simulink model "spec_Ventilation"  (R2016b)
settings: Solver=VariableStepDiscrete  StartTime=0  StopTime=100  MaxStep=1  RelTol=1e-3  EnableMultiTasking=on
libraries: carnot x6, simulink x1
settings Model: Creator=drhf  LastModifiedBy=drhf
settings DataIOCC: SaveFormat=Array  SignalLoggingSaveFormat=ModelDataLogs
settings OptimizationCC: ExpressionDepthLimit=2147483647  LifeSpan=inf
settings DebuggingCC: UnderspecifiedInitializationDetection=Classic  MergeDetectMultiDrivingBlocksExec=none  SolverPrmCheckMsg=warning  FcnCallInpInsideContextMsg=warning  StateNameClashWarn=warning  SFUnexpectedBacktrackingDiag=warning  SFNoUnconditionalDefaultTransitionDiag=warning  SFExecutionAtInitializationDiag=none
settings HardwareCC: ProdBitPerPointer=32  ProdBitPerSizeT=32  ProdBitPerPtrDiffT=32  ProdLargestAtomicFloat=None  ProdIntDivRoundTo=Undefined  ProdEndianess=Unspecified  ProdWordSize=32  ProdHWDeviceType=32-bit Generic
settings ModelReferenceCC: PropagateSignalLabelsOutOfModel=off
settings GRTTargetCC: TargetLangStandard=C89/C90 (ANSI)  GeneratePreprocessorConditionals=Disable all  CombineOutputUpdateFcns=off  GRTInterface=on
settings ConfigComp: CovMetricSettings=dw  CovHtmlReporting=on  CovSaveCumulativeToWorkspaceVar=on  CovSaveSingleToWorkspaceVar=on  CovExternalEMLEnable=off

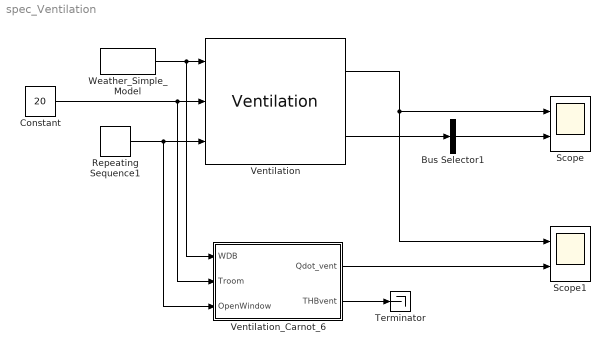
== system spec_Ventilation ==
  Bus Selector1 : BusSelector  OutputSignals=MassFlow  OutputAsBus=on
  Constant : Constant  Value=20
  Repeating Sequence1 : simulink/Sources/Repeating Sequence  rep_seq_t=[0 20 30 60 70 100]  rep_seq_y="[0  0  1   1   0   0]"
  Scope : Scope  NumInputPorts=2
  Scope1 : Scope  NumInputPorts=2
  Terminator : Terminator
  Ventilation : carnot/Source/Ventilation/Ventilation  Ahabit=50  Hroom=2  vent=0.5  rec=0.5  ppmCO2=400  ppmVOC=0  alpha=10  H=1  W=1  Nwin=1
  Ventilation_Carnot_6 : Subsystem  mask(Ventilation with Heat Recovery and Window){Ahabit=50, Hroom=2, vent=0.5, rec=0.5, ppmCO2=400, ppmVOC=0, alpha=10, H=1.2, W=1, Nwin=4}
      mask prompts: Ahabit "A: heated surface of the house in m²"; Hroom "H: height of room in m"; vent "Air exchange rate (volume of house per hour) in 1/h"; rec "Heat recovery of ventilation in 0..1"; ppmCO2 "Concentration of CO2 in ppm"; ppmVOC "Concentration of VOC in ppm"; alpha "maximal opening angle (°)"; H "height of window (m)"; W "width of window (m)"; Nwin "Number of windows"
      mask help:
      | Model of a mechanical ventilation system with heat recovery and a ventilation with windows.
      | The model is suitable for the simple building model (/Load/Houses/House_simpe).
      mask init:
      | rec = max(0, min(1, rec));
      mask Help: web(fullfile(path_carnot('help'),'Ventilation.html'),'-helpbrowser')
      mask TypeOptions Ahabit: Ahabit/Value
      mask TypeOptions Hroom: Hroom/Gain
      mask TypeOptions vent: air_flow_rate/Gain | air_flow_rate1/Gain
      mask TypeOptions rec: heatRecovery/Value
      mask TypeOptions ppmCO2: ppmCO2/Value
      mask TypeOptions ppmVOC: ppmVOC/Value
      mask TypeOptions alpha: Window_Ventilation/alpha
      mask TypeOptions H: Window_Ventilation/H
      mask TypeOptions W: Window_Ventilation/W
      mask TypeOptions Nwin: Window_Ventilation/Nwin
      mask Display:
      | plot(0,-0.2,1.2,1.2,[0.2 0.35], [0.8 0.7])
      | plot([0.35 0.65], [0.7 0.7])
      | plot([0.65 0.8], [0.7 0.8])
      | plot([0.65 0.8], [0.76 0.8])
      | plot([0.7 0.8], [0.65 0.8])
      | 
      | plot([0.2 0.35], [0.2 0.3])
      | plot([0.35 0.65], [0.3 0.3])
      | plot([0.65 0.8], [0.3 0.2])
      | plot([0.2 0.25], [0.2 0.32])
      | plot([0.2 0.35], [0.2 0.23])
      | 
      | plot ([0.45 0.45], [0 1])
      | plot ([0.55 0.55], [0 1])
      | 
      | plot ([0.45 0.55], [0.2 0.2])
      | plot ([0.45 0.55], [0.8 0.8])
      | 
      | plot ([0.45 0.55], [0 0.2])
      | plot ([0.45 0.55], [0.8 1])
  Weather_Simple_Model : carnot/Weather/Weather_Simple_Model  lat=60  Ibn=900  Idg=100  tamb=0  deltaTsky=-6  rh=50  precip="10e-3/24/3600           % 10 mm in 24 h"  cloud=0.125  p=1013e2  vw=1  wdir=270
  wires:
  Ventilation/1 -> Scope1/1, Scope/1
  Constant/1 -> Ventilation_Carnot_6/2(Troom), Ventilation/2
  Repeating Sequence1/1 -> Ventilation_Carnot_6/3(OpenWindow), Ventilation/3
  Ventilation/2 -> Bus Selector1/1
  Weather_Simple_Model/1 -> Ventilation_Carnot_6/1(WDB), Ventilation/1
  Bus Selector1/1 -> Scope/2
  Ventilation_Carnot_6/1(Qdot_vent) -> Scope1/2
  Ventilation_Carnot_6/2(THBvent) -> Terminator/1

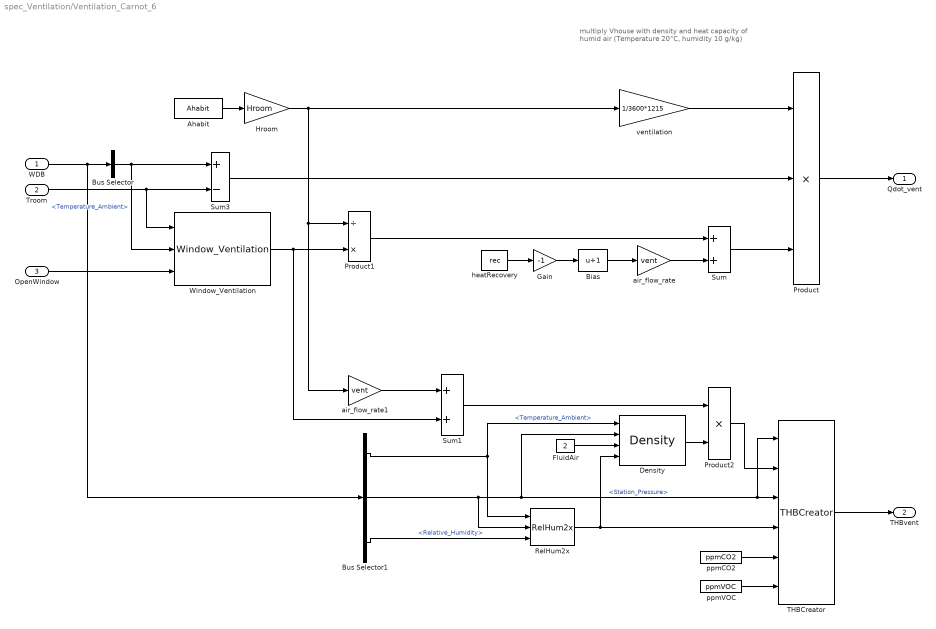
== system spec_Ventilation/Ventilation_Carnot_6 ==
  note: multiply Vhouse with
      | density and heat capacity of humid air
      | (Temperature 20°C, humidity 10 g/kg)
  WDB : Inport
  Troom : Inport  Port=2
  OpenWindow : Inport  Port=3
  Ahabit : Constant  Value=Ahabit
  Bias : Bias  Bias=1
  Bus Selector : BusSelector  OutputSignals=Temperature_Ambient
  Bus Selector1 : BusSelector  OutputSignals=Temperature_Ambient,Station_Pressure,Relative_Humidity
  Density : carnot/Basic/Material_Properties/Density  VariantControl=CarlibClassic  INPUTARGUMENTS=state variables (classic)  DEBUGLEVEL=DEBUGLEVEL  MAXTOTALWARNINGS=inf  MAXCONSECUTIVEWARNINGS=inf  WRITETOFILE=0  FILENAME='errors.txt'
  FluidAir : Constant  Value=2
  Gain : Gain  Gain=-1
  Hroom : Gain  Gain=Hroom
  Product : Product  Inputs=3  RndMeth=Zero
  Product1 : Product  Inputs=/*  RndMeth=Zero
  Product2 : Product  RndMeth=Zero
  RelHum2x : carnot/Basic/Material_Properties/RelHum2x
  Sum : Sum
  Sum1 : Sum
  Sum3 : Sum  Inputs=+-  SaturateOnIntegerOverflow=on  InputSameDT=on  OutDataTypeStr=Inherit: Same as first input
  THBCreator : carnot/Basic/Hydraulics/THBCreator  Inport_ID=off  Inport_T=on  Inport_mdot=on  Inport_p=on  Inport_type=off  Inport_mix=on  Inport_mix2=on  Inport_mix3=on  Inport_d=off  Inport_c=off  Inport_l=off  Inport_q=off  Inport_LH=off  Inport_H=off  ID=1  T=20  mdot=0  p=1e5  FluidType=2  FluidMix=0  FluidMix2=0  FluidMix3=0  d=1  c=0  l=0  q=0  LH=1  H=0  Annotation_ID=off  Annotation_T=off  Annotation_mdot=off  Annotation_p=off  Annotation_type=off  Annotation_mix=off  Annotation_mix2=off  Annotation_mix3=off  Annotation_d=off  Annotation_c=off  Annotation_l=off  Annotation_q=off  Annotation_LH=off  Annotation_H=off
  Window_Ventilation : carnot/Source/Ventilation/Window_Ventilation  alpha=alpha  H=H  W=W  Nwin=Nwin
  air_flow_rate : Gain  Gain=vent
  air_flow_rate1 : Gain  Gain=vent
  heatRecovery : Constant  Value=rec
  ppmCO2 : Constant  Value=ppmCO2
  ppmVOC : Constant  Value=ppmVOC
  ventilation : Gain  Gain=1/3600*1215  SaturateOnIntegerOverflow=on  OutDataTypeStr=Inherit: Same as input  ParamDataTypeStr=Inherit: Same as input
  Qdot_vent : Outport
  THBvent : Outport  Port=2
  wires:
  FluidAir/1 -> Density/3
  Density/1 -> Product2/2
  Sum1/1 -> Product2/1
  air_flow_rate1/1 -> Sum1/1
  Product2/1 -> THBCreator/2
  ppmVOC/1 -> THBCreator/6
  ppmCO2/1 -> THBCreator/5
  RelHum2x/1 -> THBCreator/4, Density/4
  Bus Selector1/3 -> RelHum2x/3  "<Relative_Humidity>"
  Bus Selector1/2 -> RelHum2x/2, Density/2, THBCreator/3, THBCreator/1  "<Station_Pressure>"
  Bus Selector1/1 -> RelHum2x/1, Density/1  "<Temperature_Ambient>"
  Bus Selector/1 -> Window_Ventilation/2, Sum3/1  "<Temperature_Ambient>"
  THBCreator/1 -> THBvent/1
  Window_Ventilation/1 -> Product1/2, Sum1/2
  Sum/1 -> Product/3
  Product/1 -> Qdot_vent/1
  Ahabit/1 -> Hroom/1
  ventilation/1 -> Product/1
  Sum3/1 -> Product/2
  WDB/1 -> Bus Selector1/1, Bus Selector/1
  Product1/1 -> Sum/1
  Troom/1 -> Window_Ventilation/1, Sum3/2
  OpenWindow/1 -> Window_Ventilation/3
  heatRecovery/1 -> Gain/1
  Gain/1 -> Bias/1
  Bias/1 -> air_flow_rate/1
  air_flow_rate/1 -> Sum/2
  Hroom/1 -> Product1/1, air_flow_rate1/1, ventilation/1
